simulink library "RoombaSimulink"  (R2017b)
settings: Solver=VariableStepAuto  StartTime=0.0  StopTime=10.0  RelTol=1e-3
libraries: Alarm_Library x1, Sensor_Wheellib x1
settings Model: Creator=Mark  LastModifiedBy=segadiallo

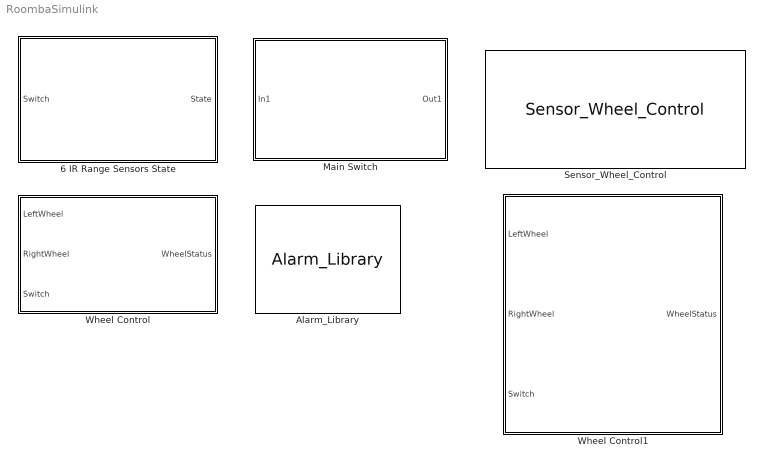
== system RoombaSimulink ==
  6 IR Range Sensors State : Subsystem  mask(Sensor Read){}
      mask help:
      | Input 0 to turn off block
      | Input 1 to turn on block
      mask Display:
      | disp('IR Sensors State')
      | port_label('input',1,'Control')
      | port_label('output',1,'State')
  Alarm_Library : Alarm_Library/Alarm_Library  SystemSampleTime=-1
  Main Switch : Subsystem
      mask help:
      | Input 0 to turn off the system
      | Input 1 to turn on the system
      mask Display:
      | disp('Main Switch')
      | port_label('input',1,'Input')
      | port_label('output',1,'Control')
  Sensor_Wheel_Control : Sensor_Wheellib/Sensor_Wheel_Control  v0=0.2
  Wheel Control : Subsystem  mask(Control){}
      mask help:
      | Input -0.5~0.5 to LeftWheel and RightWheel to control the two wheels independently.
      | Switch: input 0 to turn off block; input 1 to turn on block; input 2 to pause wheel motions.
      mask Display:
      | disp('Wheel Control')
      | port_label('input',1,'LeftWheel')
      | port_label('input',2,'RightWheel')
      | port_label('input',3,'Control')
      | port_label('output',1,'Status')
      | %port_label('input',4,'Break')
  Wheel Control1 : Subsystem  AncestorBlock=RoombaSimulink/Wheel Control  mask(Control){}
      mask help:
      | Input -0.5~0.5 to LeftWheel and RightWheel to control the two wheels independently.
      | Switch: input 0 to turn off block; input 1 to turn on block; input 2 to pause wheel motions.
      mask Display:
      | disp('Wheel Control')
      | port_label('input',1,'LeftWheel')
      | port_label('input',2,'RightWheel')
      | port_label('input',3,'Control')
      | port_label('output',1,'Status')
      | %port_label('input',4,'Break')

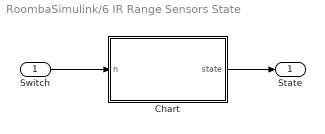
== system RoombaSimulink/6 IR Range Sensors State ==
  Switch : Inport
  Chart : Stateflow chart  TreatAsAtomicUnit=on
  "State " : Outport
  wires:
  Chart/1(state) -> "State "/1
  Switch/1 -> Chart/1(n)

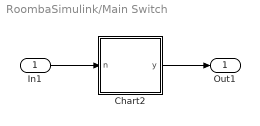
== system RoombaSimulink/Main Switch ==
  In1 : Inport
  Chart2 : Stateflow chart  TreatAsAtomicUnit=on
  Out1 : Outport
  wires:
  Chart2/1(y) -> Out1/1
  In1/1 -> Chart2/1(n)

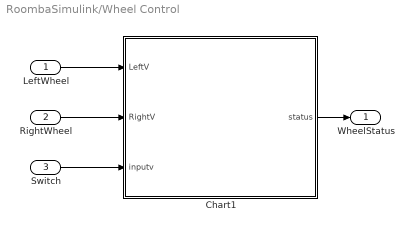
== system RoombaSimulink/Wheel Control ==
  LeftWheel : Inport
  RightWheel : Inport  Port=2
  Switch : Inport  Port=3
  Chart1 : Stateflow chart  TreatAsAtomicUnit=on
  WheelStatus : Outport
  wires:
  LeftWheel/1 -> Chart1/1(LeftV)
  Chart1/1(status) -> WheelStatus/1
  RightWheel/1 -> Chart1/2(RightV)
  Switch/1 -> Chart1/3(inputv)

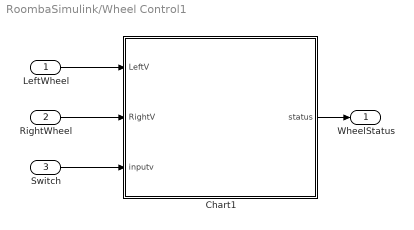
== system RoombaSimulink/Wheel Control1 ==
  LeftWheel : Inport
  RightWheel : Inport  Port=2
  Switch : Inport  Port=3
  Chart1 : Stateflow chart  TreatAsAtomicUnit=on
  WheelStatus : Outport
  wires:
  LeftWheel/1 -> Chart1/1(LeftV)
  Chart1/1(status) -> WheelStatus/1
  RightWheel/1 -> Chart1/2(RightV)
  Switch/1 -> Chart1/3(inputv)

== stateflow chart RoombaSimulink/Wheel Control/Chart1 ==
  state START
    entry: status=0
  state Connect
    entry: coder.extrinsic('evalin')
    so=evalin('base','objWs')
  state Update
  state Run
    entry:
    coder.extrinsic('SetWheelVelRoomba')
    SetWheelVelRoomba(so,RightV, LeftV)
    status=1
  state Off
    %entry: fclose(so);
    entry:  status=0
  state Pause [commented out]
    entry:
    coder.extrinsic('SetWheelVelRoomba')
    SetWheelVelRoomba(so,0, 0)
    status=2
  (default) -> START
  Off -> Connect : [inputv==2]
  START -> Connect : [inputv==2]
  Connect -> Run [order 2] : [inputv==2]
  Connect -> Off [order 1] : [inputv==0]
  Update -> Run : after(0.5,sec)
  Run -> Update [order 1] : [inputv==2]
  Run -> Off [order 2] : [inputv==0]
  Pause -> Run [commented out] : [break0==0]
  Run -> Pause [commented out] : [break0==1]
  Pause -> Off [commented out] : [inputv==0]
  data: LeftV input; RightV input; inputv input; status output; so local

== stateflow chart RoombaSimulink/Main Switch/Chart2 ==
  state START
    entry: y=0
  state CONNECT
    entry: tcpInit;
  state DISCONNECT
    entry: y=0
    coder.extrinsic('evalin')
    so=evalin('base','objWs')
    fclose(so)
  state INcrement
    entry: y = y + 1
    if y==3
    y=1
    end
  state SerialControl1
    entry: y==1
  (default) -> START
  START -> CONNECT : [n==1]
  DISCONNECT -> CONNECT : [n==1]
  CONNECT -> DISCONNECT [order 1] : [n==0]
  SerialControl1 -> DISCONNECT [order 2] : [n==0]
  CONNECT -> SerialControl1 [order 2]
  INcrement -> SerialControl1 : after(1,sec)
  SerialControl1 -> INcrement [order 1] : [n==1]
  data: n input; y output; so local
  function tcpInit:
    | function tcpInit
    | coder.extrinsic('tcpip');
    | coder.extrinsic('assignin');
    | persistent obj
    | if isempty(obj)
    |     obj=tcpip('10.0.0.1',9001);
    |     assignin('base','objWs',obj);
    |  
    |     set(obj,'Terminator','LF');
    | set(obj,'InputBufferSize',1000)
    | set(obj, 'Timeout', .5)
    | set(obj, 'ByteOrder','bigEndian');
    | 
    |  
    |  fopen(obj);
    |  
    |  fwrite(obj,128);
    | pause(.1)
    | 
    | fwrite(obj,132);
    | pause(.1)
    | 
    | % %Print 'go' on display
    | fwrite(obj, [164, 71, 79, 32, 32]);
    | % make a sound
    | fwrite(obj, [140 1 3 60 20 72 20 84 40 ]); %RoombaInit Song
    | fwrite(obj, [140 2 1 60 20]); % BeepRoomba song
    | fwrite(obj, [140 3 3 84 20 72 30 60 40]); % PowerOffRoomba song
    | fwrite(obj, [141 1]); % play RoombaInit song
    | pause(1);
    | so=obj;
    | end

== stateflow chart RoombaSimulink/6 IR Range Sensors State/Chart ==
  state CONNECT
    entry: coder.extrinsic('evalin')
    so=evalin('base','objWs')
  state START
    entry: state=[nan;nan;nan;nan;nan;nan;]
  state READ
    entry,du:
    coder.extrinsic('evalin')
    so=evalin('base','objWs')
    coder.extrinsic('RangeStateRoomba')
    state=RangeStateRoomba(so)
  state TRUNOFF
    %entry: fclose(so)
    entry:  state=[nan;nan;nan;nan;nan;nan;]
  (default) -> START
  START -> CONNECT : [n==1]
  CONNECT -> READ
  TRUNOFF -> CONNECT : [n==1]
  READ -> TRUNOFF : [n==0]
  data: state output double size=6; n input; so local

== stateflow chart RoombaSimulink/Wheel Control1/Chart1 ==
  state START
    entry: status=0
  state Connect
    entry: coder.extrinsic('evalin')
    so=evalin('base','objWs')
  state Run
    entry,du:
    coder.extrinsic('SetWheelVelRoomba')
    SetWheelVelRoomba(so,RightV, LeftV)
    status=1
  state Off
    %entry: fclose(so);
    entry:  status=0
  state Pause [commented out]
    entry:
    coder.extrinsic('SetWheelVelRoomba')
    SetWheelVelRoomba(so,0, 0)
    status=2
  (default) -> START
  Off -> Connect : [inputv==4]
  START -> Connect : [inputv==4]
  Connect -> Run [order 2] : [inputv==2]
  Connect -> Off [order 1] : [inputv==0]
  Run -> Off : [inputv==0]
  Pause -> Run [commented out] : [break0==0]
  Run -> Pause [commented out] : [break0==1]
  Pause -> Off [commented out] : [inputv==0]
  data: LeftV input; RightV input; inputv input; status output; so local
